simulink model "lqrRoll"  (R2020a)
settings: Solver=VariableStepAuto  StartTime=0.0  StopTime=40  RelTol=1e-3
values from neighbouring files (symbols this model uses):
  Alat = [0 1 0 0 0 ... (first row only)    [b747_dynInv_lat.m]
  Blat = Blat(:,2)    [b747_dynInv_lat.m]
  Clat = eye(5)    [b747_dynInv_lat.m]
  Dlat = zeros(size(Clat,1),size(Blat,2))    [b747_dynInv_lat.m]
  kd = 1.5    [b747_dynInv_lat.m]
  ki = 1.9    [b747_dynInv_lat.m]
  kLQR = lqr(Alat,Blat,Q,R)    [b747_dynInv_lat.m]
  kp = 5    [b747_dynInv_lat.m]
libraries: simulink_extras x16, simulink x2
settings Model: Creator=aaron  LastModifiedBy=aaron

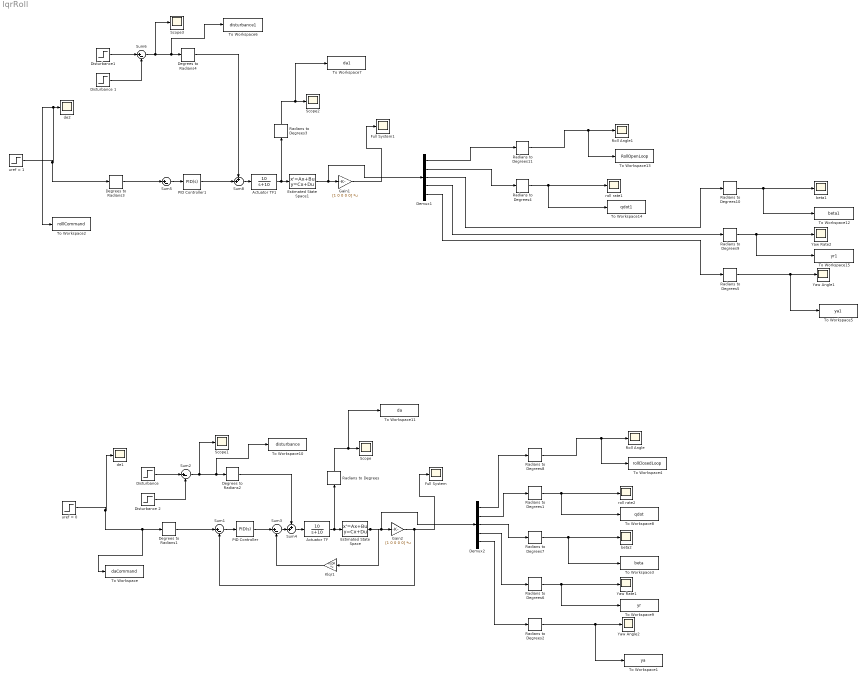
== system lqrRoll ==
  Actuator TF : TransferFcn  Numerator=[10]  Denominator=[1 10]
  Actuator TF1 : TransferFcn  Numerator=[10]  Denominator=[1 10]
  Degrees to Radians{1..4} (4 alike) : simulink_extras/Transformations/Degrees to Radians
  Demux1 : Demux  Outputs=5
  Demux2 : Demux  Outputs=5
  Disturbance : Step  Time=5  After=20  SampleTime=0
  Disturbance 1 : Step  Time=7  After=20  SampleTime=0
  Disturbance 2 : Step  Time=7  After=20  SampleTime=0
  Disturbance1 : Step  Time=5  After=20  SampleTime=0
  Estimated State Space : StateSpace  A=Alat  B=Blat  C=Clat  D=Dlat  InitialCondition=0  ContinuousStateAttributes='OpenLoop'
  Estimated State Space1 : StateSpace  A=Alat  B=Blat  C=Clat  D=Dlat  InitialCondition=0  ContinuousStateAttributes='OpenLoop'
  Full System : Scope
  Full System1 : Scope
  Gain1 : Gain  Gain=[1 0 0 0 0]  Multiplication=Matrix(K*u)
  Gain2 : Gain  Gain=[1 0 0 0 0]  Multiplication=Matrix(K*u)
  Klqr1 : Gain  Gain=kLQR  Multiplication=Matrix(K*u)
  PID Controller : simulink/Continuous/PID Controller  Controller=PID  Form=Parallel  TimeDomain=Continuous-time  UseExternalTs=off  SampleTime=-1  IntegratorMethod=Forward Euler  FilterMethod=Forward Euler  ControllerParametersSource=internal  P=kp  I=ki  D=kd  UseFilter=on  N=100  TunerSelectOption=Frequency Response Based  InitialConditionSource=internal  InitialConditionForIntegrator=0  InitialConditionForFilter=0  DifferentiatorICPrevScaledInput=0  ExternalReset=none  TrackingMode=off  Kt=1  LimitOutput=off  UpperSaturationLimit=inf  LowerSaturationLimit=-inf  LinearizeAsGain=on  AntiWindupMode=none  Kb=1  POutMin=[]  POutMax=[]  IOutMin=[]  IOutMax=[]  DOutMin=[]  DOutMax=[]  NOutMin=[]  NOutMax=[]  SumOutMin=[]  SumOutMax=[]  SaturationOutMin=[]  SaturationOutMax=[]  PParamMin=[]  PParamMax=[]  IParamMin=[]  IParamMax=[]  DParamMin=[]  DParamMax=[]  NParamMin=[]  NParamMax=[]  KbParamMin=[]  KbParamMax=[]  KtParamMin=[]  KtParamMax=[]  KbOutMin=[]  KbOutMax=[]  KtOutMin=[]  KtOutMax=[]  IntegratorOutMin=[]  IntegratorOutMax=[]  FilterOutMin=[]  FilterOutMax=[]  SumI1OutMin=[]  SumI1OutMax=[]  SumI2OutMin=[]  SumI2OutMax=[]  SumI3OutMin=[]  SumI3OutMax=[]  SumI4OutMin=[]  SumI4OutMax=[]  SumDOutMin=[]  SumDOutMax=[]  DifferentiatorOutMin=[]  DifferentiatorOutMax=[]  FilterDiffOutCoefMin=[]  FilterDiffOutCoefMax=[]  ReciprocalOutMin=[]  ReciprocalOutMax=[]  SumDenOutMin=[]  SumDenOutMax=[]  SumNumOutMin=[]  SumNumOutMax=[]  DivideOutMin=[]  DivideOutMax=[]  UdiffTsProdOutMin=[]  UdiffTsProdOutMax=[]  NTsProdOutMin=[]  NTsProdOutMax=[]  UintegralTsProdOutMin=[]  UintegralTsProdOutMax=[]  UngainTsProdOutMin=[]  UngainTsProdOutMax=[]  IntegratorContinuousStateAttributes=''  IntegratorStateMustResolveToSignalObject=off  IntegratorRTWStateStorageClass=Auto  FilterContinuousStateAttributes=''  FilterStateMustResolveToSignalObject=off  FilterRTWStateStorageClass=Auto  ParallelPVariant=InternalParameters  IdealPVariant=Disabled  IVariant=InternalParameters  DVariant=InternalParameters  IntegratorVariant=Continuous  SatVariant=Disabled  AWVariant=Passthrough  PCopyVariant=Disabled  TRVariant=Disabled  FdbkBlocksVariant=Forward  IdealPFdbkVariant=Disabled  SatFdbkVariant=Disabled  DerivativeFilterVariant=ContFilter  NVariant=InternalParameters  NCopyVariant=Disabled  FilterICVariant=InternalICsFilter  IntegratorICVariant=InternalICs  ExternalResetVariant=Disabled  TRSumVariant=Passthrough  SumFdbkVariant=Disabled  SumVariant=Sum_PID  TsampFilterVariant=InternalTs  TsampNgainVariant=Passthrough  TsampIntegralVariant=Passthrough
  PID Controller1 : simulink/Continuous/PID Controller  Controller=PID  Form=Parallel  TimeDomain=Continuous-time  UseExternalTs=off  SampleTime=-1  IntegratorMethod=Forward Euler  FilterMethod=Forward Euler  ControllerParametersSource=internal  P=5  I=1.9  D=1.5  UseFilter=on  N=100  TunerSelectOption=Frequency Response Based  InitialConditionSource=internal  InitialConditionForIntegrator=0  InitialConditionForFilter=0  DifferentiatorICPrevScaledInput=0  ExternalReset=none  TrackingMode=off  Kt=1  LimitOutput=off  UpperSaturationLimit=inf  LowerSaturationLimit=-inf  LinearizeAsGain=on  AntiWindupMode=none  Kb=1  POutMin=[]  POutMax=[]  IOutMin=[]  IOutMax=[]  DOutMin=[]  DOutMax=[]  NOutMin=[]  NOutMax=[]  SumOutMin=[]  SumOutMax=[]  SaturationOutMin=[]  SaturationOutMax=[]  PParamMin=[]  PParamMax=[]  IParamMin=[]  IParamMax=[]  DParamMin=[]  DParamMax=[]  NParamMin=[]  NParamMax=[]  KbParamMin=[]  KbParamMax=[]  KtParamMin=[]  KtParamMax=[]  KbOutMin=[]  KbOutMax=[]  KtOutMin=[]  KtOutMax=[]  IntegratorOutMin=[]  IntegratorOutMax=[]  FilterOutMin=[]  FilterOutMax=[]  SumI1OutMin=[]  SumI1OutMax=[]  SumI2OutMin=[]  SumI2OutMax=[]  SumI3OutMin=[]  SumI3OutMax=[]  SumI4OutMin=[]  SumI4OutMax=[]  SumDOutMin=[]  SumDOutMax=[]  DifferentiatorOutMin=[]  DifferentiatorOutMax=[]  FilterDiffOutCoefMin=[]  FilterDiffOutCoefMax=[]  ReciprocalOutMin=[]  ReciprocalOutMax=[]  SumDenOutMin=[]  SumDenOutMax=[]  SumNumOutMin=[]  SumNumOutMax=[]  DivideOutMin=[]  DivideOutMax=[]  UdiffTsProdOutMin=[]  UdiffTsProdOutMax=[]  NTsProdOutMin=[]  NTsProdOutMax=[]  UintegralTsProdOutMin=[]  UintegralTsProdOutMax=[]  UngainTsProdOutMin=[]  UngainTsProdOutMax=[]  IntegratorContinuousStateAttributes=''  IntegratorStateMustResolveToSignalObject=off  IntegratorRTWStateStorageClass=Auto  FilterContinuousStateAttributes=''  FilterStateMustResolveToSignalObject=off  FilterRTWStateStorageClass=Auto  ParallelPVariant=InternalParameters  IdealPVariant=Disabled  IVariant=InternalParameters  DVariant=InternalParameters  IntegratorVariant=Continuous  SatVariant=Disabled  AWVariant=Passthrough  PCopyVariant=Disabled  TRVariant=Disabled  FdbkBlocksVariant=Forward  IdealPFdbkVariant=Disabled  SatFdbkVariant=Disabled  DerivativeFilterVariant=ContFilter  NVariant=InternalParameters  NCopyVariant=Disabled  FilterICVariant=InternalICsFilter  IntegratorICVariant=InternalICs  ExternalResetVariant=Disabled  TRSumVariant=Passthrough  SumFdbkVariant=Disabled  SumVariant=Sum_PID  TsampFilterVariant=InternalTs  TsampNgainVariant=Passthrough  TsampIntegralVariant=Passthrough
  Radians to Degrees{,1..11} (12 alike) : simulink_extras/Transformations/Radians to Degrees
  Roll Angle : Scope
  Roll Angle1 : Scope
  Scope{,1..3} (4 alike) : Scope
  Sum{1..3,5..6} (5 alike) : Sum  Inputs=|+-
  Sum4 : Sum  Inputs=++|
  Sum8 : Sum  Inputs=++|
  To Workspace : ToWorkspace  VariableName=daCommand  SampleTime=-1
  To Workspace1 : ToWorkspace  VariableName=ya  SampleTime=-1
  To Workspace10 : ToWorkspace  VariableName=disturbance  SampleTime=-1
  To Workspace11 : ToWorkspace  VariableName=da  SampleTime=-1
  To Workspace12 : ToWorkspace  VariableName=beta1  SampleTime=-1
  To Workspace13 : ToWorkspace  VariableName=RollOpenLoop  SampleTime=-1
  To Workspace14 : ToWorkspace  VariableName=qdot1  SampleTime=-1
  To Workspace15 : ToWorkspace  VariableName=yr1  SampleTime=-1
  To Workspace2 : ToWorkspace  VariableName=rolllCommand  SampleTime=-1
  To Workspace3 : ToWorkspace  VariableName=beta  SampleTime=-1
  To Workspace4 : ToWorkspace  VariableName=rollClosedLoop  SampleTime=-1
  To Workspace5 : ToWorkspace  VariableName=ya1  SampleTime=-1
  To Workspace6 : ToWorkspace  VariableName=disturbance1  SampleTime=-1
  To Workspace7 : ToWorkspace  VariableName=da1  SampleTime=-1
  To Workspace8 : ToWorkspace  VariableName=qdot  SampleTime=-1
  To Workspace9 : ToWorkspace  VariableName=yr  SampleTime=-1
  Yaw Angle1 : Scope
  Yaw Angle2 : Scope
  Yaw Rate1 : Scope
  Yaw Rate2 : Scope
  beta1 : Scope
  beta2 : Scope
  de1 : Scope
  de2 : Scope
  roll rate1 : Scope
  roll rate2 : Scope
  uref = 0 : Step  After=0  SampleTime=0
  uref = 1 : Step  After=0  SampleTime=0
  wires:
  Demux2/5 -> Radians to Degrees2/1
  Radians to Degrees7/1 -> To Workspace3/1, beta2/1
  Demux2/4 -> Radians to Degrees6/1
  Demux2/2 -> Radians to Degrees1/1
  Radians to Degrees6/1 -> To Workspace9/1, Yaw Rate1/1
  Klqr1/1 -> Sum3/2
  Radians to Degrees8/1 -> Roll Angle/1, To Workspace4/1
  Demux2/3 -> Radians to Degrees7/1
  Demux2/1 -> Radians to Degrees8/1
  Radians to Degrees2/1 -> To Workspace1/1, Yaw Angle2/1
  Radians to Degrees1/1 -> To Workspace8/1, roll rate2/1
  Estimated State Space/1 -> Demux2/1, Gain2/1, Klqr1/1
  Gain2/1 -> Full System/1, Sum1/2
  Degrees to Radians1/1 -> Sum1/1
  PID Controller/1 -> Sum3/1
  Actuator TF/1 -> Estimated State Space/1, Radians to Degrees/1
  Sum2/1 -> Scope1/1, To Workspace10/1, Degrees to Radians2/1
  Disturbance 2/1 -> Sum2/2
  Disturbance/1 -> Sum2/1
  Sum1/1 -> PID Controller/1
  Sum4/1 -> Actuator TF/1
  Degrees to Radians2/1 -> Sum4/1
  Sum3/1 -> Sum4/2
  Radians to Degrees/1 -> To Workspace11/1, Scope/1
  uref = 0/1 -> To Workspace/1, Degrees to Radians1/1, de1/1
  Radians to Degrees3/1 -> To Workspace7/1, Scope2/1
  Demux1/3 -> Radians to Degrees10/1
  Radians to Degrees11/1 -> Roll Angle1/1, To Workspace13/1
  Demux1/4 -> Radians to Degrees9/1
  uref = 1/1 -> Degrees to Radians3/1, To Workspace2/1, de2/1
  Radians to Degrees9/1 -> To Workspace15/1, Yaw Rate2/1
  Radians to Degrees10/1 -> To Workspace12/1, beta1/1
  Demux1/5 -> Radians to Degrees5/1
  Demux1/2 -> Radians to Degrees4/1
  Degrees to Radians3/1 -> Sum5/1
  Estimated State Space1/1 -> Demux1/1, Gain1/1
  Radians to Degrees5/1 -> To Workspace5/1, Yaw Angle1/1
  Demux1/1 -> Radians to Degrees11/1
  Degrees to Radians4/1 -> Sum8/1
  Sum5/1 -> PID Controller1/1
  Radians to Degrees4/1 -> To Workspace14/1, roll rate1/1
  Gain1/1 -> Full System1/1
  Sum8/1 -> Actuator TF1/1
  PID Controller1/1 -> Sum8/2
  Sum6/1 -> Scope3/1, To Workspace6/1, Degrees to Radians4/1
  Disturbance 1/1 -> Sum6/2
  Actuator TF1/1 -> Estimated State Space1/1, Radians to Degrees3/1
  Disturbance1/1 -> Sum6/1
